simulink model "chap05"  (R2021a)
settings: Solver=FixedStepDiscrete  StartTime=0.0  StopTime=inf  FixedStep=0.001  RelTol=1e-3
undefined symbols (not defined in the file): DiscIntNeverNeededParam, Header, Pose, X, Y, Z
libraries: robotlib x31
(part 3 of 9)

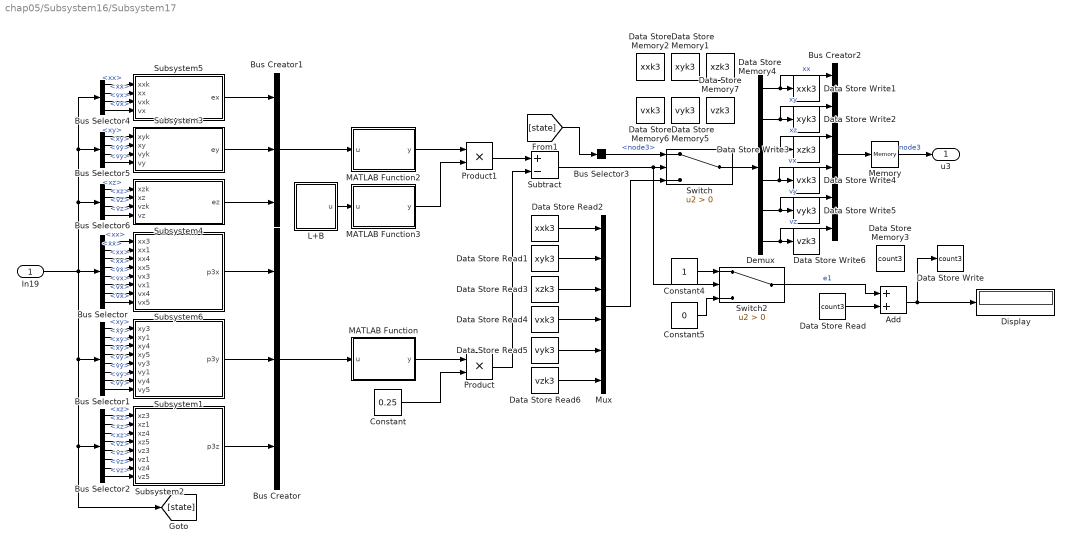
== system chap05/Subsystem16/Subsystem17 ==
  In19 : Inport
  Add : Sum
  Bus Creator : BusCreator  Inputs=3
  Bus Creator1 : BusCreator  Inputs=3
  Bus Creator2 : BusCreator  Inputs=6
  Bus Selector : BusSelector  OutputSignals=state(tk).node3.xx,state(tk).node1.xx,state(tk).node4.xx,state(tk).node5.xx,state(tk).node3.vx,state(tk).node1.vx,state(tk).node4.vx,state(tk).node5.vx
  Bus Selector1 : BusSelector  OutputSignals=state(tk).node3.xy,state(tk).node1.xy,state(tk).node4.xy,state(tk).node5.xy,state(tk).node3.vy,state(tk).node1.vy,state(tk).node4.vy,state(tk).node5.vy
  Bus Selector2 : BusSelector  OutputSignals=state(tk).node3.xz,state(tk).node1.xz,state(tk).node4.xz,state(tk).node5.xz,state(tk).node3.vz,state(tk).node1.vz,state(tk).node4.vz,state(tk).node5.vz
  Bus Selector3 : BusSelector  OutputSignals=state(t).node3
  Bus Selector4 : BusSelector  OutputSignals=state(tk).node3.xx,state(t).node3.xx,state(tk).node3.vx,state(t).node3.vx
  Bus Selector5 : BusSelector  OutputSignals=state(tk).node3.xy,state(t).node3.xy,state(tk).node3.vy,state(t).node3.vy
  Bus Selector6 : BusSelector  OutputSignals=state(tk).node3.xz,state(t).node3.xz,state(tk).node3.vz,state(t).node3.vz
  Constant : Constant  Value=0.25
  Constant4 : Constant
  Constant5 : Constant  Value=0
  Data Store Memory1 : DataStoreMemory  DataStoreName=xyk3  ReadBeforeWriteMsg=warning  WriteAfterWriteMsg=warning  WriteAfterReadMsg=warning  ShowAdditionalParam=off
  Data Store Memory2 : DataStoreMemory  DataStoreName=xxk3  ReadBeforeWriteMsg=warning  WriteAfterWriteMsg=warning  WriteAfterReadMsg=warning  ShowAdditionalParam=off
  Data Store Memory3 : DataStoreMemory  DataStoreName=count3  ReadBeforeWriteMsg=warning  WriteAfterWriteMsg=warning  WriteAfterReadMsg=warning  ShowAdditionalParam=off
  Data Store Memory4 : DataStoreMemory  DataStoreName=xzk3  ReadBeforeWriteMsg=warning  WriteAfterWriteMsg=warning  WriteAfterReadMsg=warning  ShowAdditionalParam=off
  Data Store Memory5 : DataStoreMemory  DataStoreName=vyk3  ReadBeforeWriteMsg=warning  WriteAfterWriteMsg=warning  WriteAfterReadMsg=warning  ShowAdditionalParam=off
  Data Store Memory6 : DataStoreMemory  DataStoreName=vxk3  ReadBeforeWriteMsg=warning  WriteAfterWriteMsg=warning  WriteAfterReadMsg=warning  ShowAdditionalParam=off
  Data Store Memory7 : DataStoreMemory  DataStoreName=vzk3  ReadBeforeWriteMsg=warning  WriteAfterWriteMsg=warning  WriteAfterReadMsg=warning  ShowAdditionalParam=off
  Data Store Read : DataStoreRead  DataStoreName=count3  IndexOptions=Index vector (dialog)  Indices=1  OutputSizes=1
  Data Store Read1 : DataStoreRead  DataStoreName=xyk3  IndexOptions=Index vector (dialog)  Indices=1  OutputSizes=1
  Data Store Read2 : DataStoreRead  DataStoreName=xxk3  IndexOptions=Index vector (dialog)  Indices=1  OutputSizes=1
  Data Store Read3 : DataStoreRead  DataStoreName=xzk3  IndexOptions=Index vector (dialog)  Indices=1  OutputSizes=1
  Data Store Read4 : DataStoreRead  DataStoreName=vxk3  IndexOptions=Index vector (dialog)  Indices=1  OutputSizes=1
  Data Store Read5 : DataStoreRead  DataStoreName=vyk3  IndexOptions=Index vector (dialog)  Indices=1  OutputSizes=1
  Data Store Read6 : DataStoreRead  DataStoreName=vzk3  IndexOptions=Index vector (dialog)  Indices=1  OutputSizes=1
  Data Store Write : DataStoreWrite  DataStoreName=count3  IndexOptions=Index vector (dialog)  Indices=1  OutputSizes=1
  Data Store Write1 : DataStoreWrite  DataStoreName=xxk3  IndexOptions=Index vector (dialog)  Indices=1  OutputSizes=1
  Data Store Write2 : DataStoreWrite  DataStoreName=xyk3  IndexOptions=Index vector (dialog)  Indices=1  OutputSizes=1
  Data Store Write3 : DataStoreWrite  DataStoreName=xzk3  IndexOptions=Index vector (dialog)  Indices=1  OutputSizes=1
  Data Store Write4 : DataStoreWrite  DataStoreName=vxk3  IndexOptions=Index vector (dialog)  Indices=1  OutputSizes=1
  Data Store Write5 : DataStoreWrite  DataStoreName=vyk3  IndexOptions=Index vector (dialog)  Indices=1  OutputSizes=1
  Data Store Write6 : DataStoreWrite  DataStoreName=vzk3  IndexOptions=Index vector (dialog)  Indices=1  OutputSizes=1
  Demux : Demux  Outputs=6
  Display : Display
  L+B : Subsystem
  MATLAB Function : MATLAB Function  TreatAsAtomicUnit=on
  MATLAB Function2 : MATLAB Function  TreatAsAtomicUnit=on
  MATLAB Function3 : MATLAB Function  TreatAsAtomicUnit=on
  Memory : Memory
  Mux : Mux  Inputs=6
  Product : Product
  Product1 : Product
  Subsystem1 : Subsystem
  Subsystem2 : Subsystem
  Subsystem3 : Subsystem
  Subsystem4 : Subsystem
  Subsystem5 : Subsystem
  Subsystem6 : Subsystem
  Subtract : Sum  Inputs=+-
  Switch : Switch  Criteria=u2 > Threshold
  Switch2 : Switch  Criteria=u2 > Threshold
  u3 : Outport
  wires:
  Bus Selector2/8 -> Subsystem2/8(vz5)  "<vz>"
  Bus Selector2/7 -> Subsystem2/7(vz4)  "<vz>"
  Bus Selector2/6 -> Subsystem2/6(vz1)  "<vz>"
  Bus Selector2/5 -> Subsystem2/5(vz3)  "<vz>"
  Bus Selector2/4 -> Subsystem2/4(xz5)  "<xz>"
  Bus Selector2/3 -> Subsystem2/3(xz4)  "<xz>"
  Bus Selector2/2 -> Subsystem2/2(xz1)  "<xz>"
  Bus Selector2/1 -> Subsystem2/1(xz3)  "<xz>"
  Bus Selector1/8 -> Subsystem1/8(vy5)  "<vy>"
  Bus Selector1/7 -> Subsystem1/7(vy4)  "<vy>"
  Bus Selector1/6 -> Subsystem1/6(vy1)  "<vy>"
  Bus Selector1/5 -> Subsystem1/5(vy3)  "<vy>"
  Bus Selector1/4 -> Subsystem1/4(xy5)  "<xy>"
  Bus Selector1/3 -> Subsystem1/3(xy4)  "<xy>"
  Bus Selector1/2 -> Subsystem1/2(xy1)  "<xy>"
  Bus Selector1/1 -> Subsystem1/1(xy3)  "<xy>"
  Bus Selector/8 -> Subsystem6/8(vx5)  "<vx>"
  Bus Selector/7 -> Subsystem6/7(vx4)  "<vx>"
  Bus Selector/6 -> Subsystem6/6(vx1)  "<vx>"
  Bus Selector/5 -> Subsystem6/5(vx3)  "<vx>"
  Bus Selector/4 -> Subsystem6/4(xx5)  "<xx>"
  Bus Selector/3 -> Subsystem6/3(xx4)  "<xx>"
  Bus Selector/2 -> Subsystem6/2(xx1)  "<xx>"
  Bus Selector/1 -> Subsystem6/1(xx3)  "<xx>"
  Subsystem1/1(p3y) -> Bus Creator/2
  Subsystem6/1(p3x) -> Bus Creator/1
  Subsystem2/1(p3z) -> Bus Creator/3
  Data Store Read6/1 -> Mux/6
  Switch/1 -> Demux/1
  Demux/2 -> Bus Creator2/2, Data Store Write2/1  "xy"
  Bus Selector3/1 -> Switch/1  "<node3>"
  Demux/1 -> Bus Creator2/1, Data Store Write1/1  "xx"
  Switch2/1 -> Add/1  "e1"
  Demux/6 -> Bus Creator2/6, Data Store Write6/1  "vz"
  Demux/3 -> Bus Creator2/3, Data Store Write3/1  "xz"
  Data Store Read2/1 -> Mux/1
  Constant4/1 -> Switch2/1
  Mux/1 -> Switch/3
  Data Store Read3/1 -> Mux/3
  Add/1 -> Data Store Write/1, Display/1
  Demux/4 -> Bus Creator2/4, Data Store Write4/1  "vx"
  Memory/1 -> u3/1  "node3"
  Data Store Read5/1 -> Mux/5
  Data Store Read4/1 -> Mux/4
  Product/1 -> Subtract/2
  Data Store Read1/1 -> Mux/2
  [state] -> Bus Selector3/1
  MATLAB Function3/1(y) -> Product1/2
  Bus Creator1/1 -> MATLAB Function2/1(u)
  Constant5/1 -> Switch2/3
  Constant/1 -> Product/2
  MATLAB Function2/1(y) -> Product1/1
  Subsystem4/1(ez) -> Bus Creator1/3
  Subsystem5/1(ex) -> Bus Creator1/1
  Subsystem3/1(ey) -> Bus Creator1/2
  Demux/5 -> Bus Creator2/5, Data Store Write5/1  "vy"
  Product1/1 -> Subtract/1
  Data Store Read/1 -> Add/2
  MATLAB Function/1(y) -> Product/1
  Bus Creator/1 -> MATLAB Function/1(u)
  Bus Selector6/4 -> Subsystem4/4(vz)  "<vz>"
  Bus Selector6/2 -> Subsystem4/2(xz)  "<xz>"
  Bus Selector6/3 -> Subsystem4/3(vzk)  "<vz>"
  Bus Selector6/1 -> Subsystem4/1(xzk)  "<xz>"
  Bus Selector5/3 -> Subsystem3/3(vyk)  "<vy>"
  Bus Selector5/2 -> Subsystem3/2(xy)  "<xy>"
  Bus Selector5/4 -> Subsystem3/4(vy)  "<vy>"
  Bus Selector5/1 -> Subsystem3/1(xyk)  "<xy>"
  In19/1 -> [state], Bus Selector2/1, Bus Selector1/1, Bus Selector/1, Bus Selector6/1, Bus Selector5/1, Bus Selector4/1
  Bus Selector4/1 -> Subsystem5/1(xxk)  "<xx>"
  Bus Selector4/2 -> Subsystem5/2(xx)  "<xx>"
  Bus Selector4/3 -> Subsystem5/3(vxk)  "<vx>"
  Bus Selector4/4 -> Subsystem5/4(vx)  "<vx>"
  Bus Creator2/1 -> Memory/1
  Subtract/1 -> Switch/2, Switch2/2
  L+B/1(u) -> MATLAB Function3/1(u)

== system chap05/Subsystem16/Subsystem2 ==
  In19 : Inport
  switch : Inport  Port=2
  Bus Creator : BusCreator  Inputs=3
  Bus Selector : BusSelector  OutputSignals=state(tk).node2.xx,state(tk).node1.xx,state(tk).node4.xx,state(tk).node6.xx,state(tk).node2.vx,state(tk).node1.vx,state(tk).node4.vx,state(tk).node6.vx
  Bus Selector1 : BusSelector  OutputSignals=state(tk).node2.xy,state(tk).node1.xy,state(tk).node4.xy,state(tk).node6.xy,state(tk).node2.vy,state(tk).node1.vy,state(tk).node4.vy,state(tk).node6.vy
  Bus Selector2 : BusSelector  OutputSignals=state(tk).node2.xz,state(tk).node1.xz,state(tk).node4.xz,state(tk).node6.xz,state(tk).node2.vz,state(tk).node1.vz,state(tk).node4.vz,state(tk).node6.vz
  Bus Selector3 : BusSelector  OutputSignals=state(t).node2.vx
  Bus Selector4 : BusSelector  OutputSignals=state(t).node2.vy
  Bus Selector5 : BusSelector  OutputSignals=state(t).node2.vz
  Bus Selector6 : BusSelector  OutputSignals=state(t).node2.vx,state(t).node2.vy,state(t).node2.vz
  Bus Selector7 : BusSelector  OutputSignals=state(t).node2.vx,state(t).node2.vy,state(t).node2.vz
  Bus Selector8 : BusSelector  OutputSignals=control.node2.ux,control.node2.uy,control.node2.uz
  Subsystem1 : Subsystem
  Subsystem10 : Subsystem
  Subsystem11 : Subsystem
      settings: PortSchema="{\"entries\":[{\"content\":{\"sides\":[{\"content\":{\"connectorIds\":[\"In1\",\"In2\",\"In3\"]},\"type\":\"ConnectorPlacement.EquallySpacedRectSide\",\"uuid\":\"3c32f130-2df4-4697-80e9-267a8217898e\"},{\"content\":{\"connectorIds\":[\"Out1\"],\"side\":\"RIGHT\"},\"type\":\"ConnectorPlacement.EquallySpacedRectSide\",\"uuid\":\"840675a7-4714-440f-a6ce-75eff1b2763f\"},{\"content\":{\"connectorIds\":[\"In4\"],\"side\":\"TOP\"},\"type\":\"ConnectorPlacement.EquallySpacedRectSide\",\"uuid\":\"5c23af56-4ec3-4a39-a531-12998a0be3c8\"},{\"content\":{\"connectorIds\":[\"Out2\"],\"side\":\"BOTTOM\"},\"type\":\"ConnectorPlacement.EquallySpacedRectSide\",\"uuid\":\"31d953fb-65a0-42e9-a844-060de010f298\"}]},\"type\":\"ConnectorPlacement.EquallySpacedConnector\",\"uuid\":\"61b27aa3-5880-401e-bae3-4611093a191a\"}],\"packageUris\":[\"http://schema.mathworks.com/mf0/Connector/R2020b\"],\"version\":\"1.0\"}"
  Subsystem2 : Subsystem
  Subsystem3 : Subsystem
      settings: PortSchema="{\"entries\":[{\"content\":{\"sides\":[{\"content\":{\"connectorIds\":[\"In1\",\"In2\",\"In3\",\"In4\",\"In5\",\"In6\",\"In7\",\"In8\",\"In9\"]},\"type\":\"ConnectorPlacement.EquallySpacedRectSide\",\"uuid\":\"e02b19dc-feca-4a5f-b0a9-7b682689d3dc\"},{\"content\":{\"connectorIds\":[\"Out1\",\"Out2\",\"Out3\"],\"side\":\"RIGHT\"},\"type\":\"ConnectorPlacement.EquallySpacedRectSide\",\"uuid\":\"6cba16a1-1866-4332-a766-c6ecae75c00a\"},{\"content\":{\"connectorIds\":[],\"side\":\"TOP\"},\"type\":\"ConnectorPlacement.EquallySpacedRectSide\",\"uuid\":\"834934d8-ba7c-4cfc-8528-dda956d123e9\"},{\"content\":{\"connectorIds\":[\"In10\"],\"side\":\"BOTTOM\"},\"type\":\"ConnectorPlacement.EquallySpacedRectSide\",\"uuid\":\"a447ec2e-850c-49d1-98c5-4201d925b22c\"}]},\"type\":\"ConnectorPlacement.EquallySpacedConnector\",\"uuid\":\"dde62e81-0b86-43c6-8cdc-67ebf109c079\"}],\"packageUris\":[\"http://schema.mathworks.com/mf0/Connector/R2020b\"],\"version\":\"1.0\"}"
  Subsystem4 : Subsystem
      settings: PortSchema="{\"entries\":[{\"content\":{\"sides\":[{\"content\":{\"connectorIds\":[\"In1\",\"In2\",\"In3\"]},\"type\":\"ConnectorPlacement.EquallySpacedRectSide\",\"uuid\":\"3c32f130-2df4-4697-80e9-267a8217898e\"},{\"content\":{\"connectorIds\":[\"Out1\"],\"side\":\"RIGHT\"},\"type\":\"ConnectorPlacement.EquallySpacedRectSide\",\"uuid\":\"840675a7-4714-440f-a6ce-75eff1b2763f\"},{\"content\":{\"connectorIds\":[\"In4\"],\"side\":\"TOP\"},\"type\":\"ConnectorPlacement.EquallySpacedRectSide\",\"uuid\":\"5c23af56-4ec3-4a39-a531-12998a0be3c8\"},{\"content\":{\"connectorIds\":[\"Out2\"],\"side\":\"BOTTOM\"},\"type\":\"ConnectorPlacement.EquallySpacedRectSide\",\"uuid\":\"31d953fb-65a0-42e9-a844-060de010f298\"}]},\"type\":\"ConnectorPlacement.EquallySpacedConnector\",\"uuid\":\"61b27aa3-5880-401e-bae3-4611093a191a\"}],\"packageUris\":[\"http://schema.mathworks.com/mf0/Connector/R2020b\"],\"version\":\"1.0\"}"
  Subsystem6 : Subsystem
  Subsystem8 : Subsystem
      settings: PortSchema="{\"entries\":[{\"content\":{\"sides\":[{\"content\":{\"connectorIds\":[\"In1\",\"In2\",\"In3\",\"In4\",\"In5\",\"In6\"]},\"type\":\"ConnectorPlacement.EquallySpacedRectSide\",\"uuid\":\"6e2ae49e-f829-4a88-ba6d-12a1c984ff97\"},{\"content\":{\"connectorIds\":[\"Out1\"],\"side\":\"RIGHT\"},\"type\":\"ConnectorPlacement.EquallySpacedRectSide\",\"uuid\":\"1d02df48-94d5-4b75-9fdc-37bb62799324\"},{\"content\":{\"connectorIds\":[],\"side\":\"TOP\"},\"type\":\"ConnectorPlacement.EquallySpacedRectSide\",\"uuid\":\"e0c2a01b-94eb-432a-818f-b3ac4af71c3e\"},{\"content\":{\"connectorIds\":[\"In7\"],\"side\":\"BOTTOM\"},\"type\":\"ConnectorPlacement.EquallySpacedRectSide\",\"uuid\":\"1c8c54e5-1608-4962-a210-31f0a1951aa9\"}]},\"type\":\"ConnectorPlacement.EquallySpacedConnector\",\"uuid\":\"4e183442-7783-4f10-aa1a-c21f2f9b268a\"}],\"packageUris\":[\"http://schema.mathworks.com/mf0/Connector/R2020b\"],\"version\":\"1.0\"}"
  Subsystem9 : Subsystem
      settings: PortSchema="{\"entries\":[{\"content\":{\"sides\":[{\"content\":{\"connectorIds\":[\"In1\",\"In2\",\"In3\"]},\"type\":\"ConnectorPlacement.EquallySpacedRectSide\",\"uuid\":\"3c32f130-2df4-4697-80e9-267a8217898e\"},{\"content\":{\"connectorIds\":[\"Out1\"],\"side\":\"RIGHT\"},\"type\":\"ConnectorPlacement.EquallySpacedRectSide\",\"uuid\":\"840675a7-4714-440f-a6ce-75eff1b2763f\"},{\"content\":{\"connectorIds\":[\"In4\"],\"side\":\"TOP\"},\"type\":\"ConnectorPlacement.EquallySpacedRectSide\",\"uuid\":\"5c23af56-4ec3-4a39-a531-12998a0be3c8\"},{\"content\":{\"connectorIds\":[\"Out2\"],\"side\":\"BOTTOM\"},\"type\":\"ConnectorPlacement.EquallySpacedRectSide\",\"uuid\":\"31d953fb-65a0-42e9-a844-060de010f298\"}]},\"type\":\"ConnectorPlacement.EquallySpacedConnector\",\"uuid\":\"61b27aa3-5880-401e-bae3-4611093a191a\"}],\"packageUris\":[\"http://schema.mathworks.com/mf0/Connector/R2020b\"],\"version\":\"1.0\"}"
  u2 : Outport
  wires:
  Bus Creator/1 -> u2/1  "node2"
  Bus Selector6/1 -> Subsystem8/4(vx)  "<vx>"
  Bus Selector6/2 -> Subsystem8/5(vy)  "<vy>"
  Bus Selector6/3 -> Subsystem8/6(vz)  "<vz>"
  [Sz] -> Subsystem8/3(Sz)
  [Sx] -> Subsystem8/1(Sx)
  [state] -> Bus Selector6/1
  [Sy] -> Subsystem8/2(Sy)
  Subsystem8/1(" gain") -> [gain]  "p2"
  Subsystem10/1(ux) -> Bus Creator/1  "ux"
  Subsystem10/2(uy) -> Bus Creator/2  "uy"
  Subsystem10/3(uz) -> Bus Creator/3  "uz"
  Bus Selector8/3 -> Subsystem3/8(uz)  "<uz>"
  Bus Selector7/3 -> Subsystem3/4(vz)  "<vz>"
  Bus Selector7/2 -> Subsystem3/3(vy)  "<vy>"
  Bus Selector7/1 -> Subsystem3/2(vx)  "<vx>"
  Bus Selector8/1 -> Subsystem3/6(ux)  "<ux>"
  [state] -> Bus Selector7/1
  Bus Selector8/2 -> Subsystem3/7(uy)  "<uy>"
  [state] -> Bus Selector8/1
  Subsystem3/1(udtx) -> Subsystem10/1(utx)
  Subsystem3/2(udty) -> Subsystem10/2(uty)
  Subsystem3/3(udtz) -> Subsystem10/3(utz)
  Subsystem11/2(Sz) -> [Sz]
  Subsystem9/1(uy) -> Subsystem3/5(uty)
  Subsystem1/1(p2y) -> Subsystem9/2(uty)
  [state] -> Bus Selector4/1
  Subsystem4/1(ux) -> Subsystem3/1(utx)
  Subsystem2/1(p2z) -> Subsystem11/2(utz)
  Bus Selector4/1 -> Subsystem9/1(vy2)  "<vy>"
  Bus Selector5/1 -> Subsystem11/1(vz2)  "<vz>"
  [gain] -> Subsystem11/3(gain)
  [gain] -> Subsystem4/3(gain)
  Subsystem11/1(uz) -> Subsystem3/9(utz)
  [gain] -> Subsystem9/3(gain)
  [state] -> Bus Selector3/1
  Subsystem6/1(p2x) -> Subsystem4/2(utx)
  Subsystem9/2(Sz) -> [Sy]
  Bus Selector3/1 -> Subsystem4/1(vx2)  "<vx>"
  Subsystem4/2(Sx) -> [Sx]
  [state] -> Bus Selector5/1
  In19/1 -> [state], Bus Selector2/1, Bus Selector/1, Bus Selector1/1
  Bus Selector1/6 -> Subsystem1/6(vy1)  "<vy>"
  Bus Selector2/6 -> Subsystem2/6(vz1)  "<vz>"
  Bus Selector/7 -> Subsystem6/7(vx4)  "<vx>"
  Bus Selector/3 -> Subsystem6/3(xx4)  "<xx>"
  Bus Selector1/2 -> Subsystem1/2(xy1)  "<xy>"
  Bus Selector1/5 -> Subsystem1/5(vy2)  "<vy>"
  Bus Selector/2 -> Subsystem6/2(xx1)  "<xx>"
  Bus Selector/6 -> Subsystem6/6(vx1)  "<vx>"
  Bus Selector/8 -> Subsystem6/8(vx6)  "<vx>"
  Bus Selector1/8 -> Subsystem1/8(vy6)  "<vy>"
  Bus Selector/1 -> Subsystem6/1(xx2)  "<xx>"
  Bus Selector/5 -> Subsystem6/5(vx2)  "<vx>"
  Bus Selector1/1 -> Subsystem1/1(xy2)  "<xy>"
  Bus Selector2/3 -> Subsystem2/3(xz4)  "<xz>"
  Bus Selector2/4 -> Subsystem2/4(xz6)  "<xz>"
  Bus Selector2/5 -> Subsystem2/5(vz2)  "<vz>"
  Bus Selector2/7 -> Subsystem2/7(vz4)  "<vz>"
  Bus Selector2/1 -> Subsystem2/1(xz2)  "<xz>"
  Bus Selector2/2 -> Subsystem2/2(xz1)  "<xz>"
  Bus Selector1/7 -> Subsystem1/7(vy4)  "<vy>"
  Bus Selector1/3 -> Subsystem1/3(xy4)  "<xy>"
  Bus Selector1/4 -> Subsystem1/4(xy6)  "<xy>"
  Bus Selector/4 -> Subsystem6/4(xx6)  "<xx>"
  Bus Selector2/8 -> Subsystem2/8(vz6)  "<vz>"
  switch/1 -> [switch], Subsystem4/4(switch)
  [switch] -> Subsystem9/4(switch)
  [switch] -> Subsystem11/4(switch)
  [switch] -> Subsystem3/10(switch)
  [switch] -> Subsystem8/7(switch)

== system chap05/Subsystem16/Subsystem3 ==
  In19 : Inport
  switch : Inport  Port=2
  Bus Creator : BusCreator  Inputs=3
  Bus Selector : BusSelector  OutputSignals=state(tk).node4.xx,state(tk).node2.xx,state(tk).node3.xx,state(tk).node5.xx,state(tk).node4.vx,state(tk).node2.vx,state(tk).node3.vx,state(tk).node5.vx
  Bus Selector1 : BusSelector  OutputSignals=state(tk).node4.xy,state(tk).node2.xy,state(tk).node3.xy,state(tk).node5.xy,state(tk).node4.vy,state(tk).node2.vy,state(tk).node3.vy,state(tk).node5.vy
  Bus Selector2 : BusSelector  OutputSignals=state(tk).node4.xz,state(tk).node2.xz,state(tk).node3.xz,state(tk).node5.xz,state(tk).node4.vz,state(tk).node2.vz,state(tk).node3.vz,state(tk).node5.vz
  Bus Selector3 : BusSelector  OutputSignals=state(t).node4.vx
  Bus Selector4 : BusSelector  OutputSignals=state(t).node4.vy
  Bus Selector5 : BusSelector  OutputSignals=state(t).node4.vz
  Bus Selector6 : BusSelector  OutputSignals=state(t).node4.vx,state(t).node4.vy,state(t).node4.vz
  Bus Selector7 : BusSelector  OutputSignals=state(t).node4.vx,state(t).node4.vy,state(t).node4.vz
  Bus Selector8 : BusSelector  OutputSignals=control.node4.ux,control.node4.uy,control.node4.uz
  Subsystem1 : Subsystem
  Subsystem10 : Subsystem
  Subsystem11 : Subsystem
      settings: PortSchema="{\"entries\":[{\"content\":{\"sides\":[{\"content\":{\"connectorIds\":[\"In1\",\"In2\",\"In3\"]},\"type\":\"ConnectorPlacement.EquallySpacedRectSide\",\"uuid\":\"3c32f130-2df4-4697-80e9-267a8217898e\"},{\"content\":{\"connectorIds\":[\"Out1\"],\"side\":\"RIGHT\"},\"type\":\"ConnectorPlacement.EquallySpacedRectSide\",\"uuid\":\"840675a7-4714-440f-a6ce-75eff1b2763f\"},{\"content\":{\"connectorIds\":[\"In4\"],\"side\":\"TOP\"},\"type\":\"ConnectorPlacement.EquallySpacedRectSide\",\"uuid\":\"5c23af56-4ec3-4a39-a531-12998a0be3c8\"},{\"content\":{\"connectorIds\":[\"Out2\"],\"side\":\"BOTTOM\"},\"type\":\"ConnectorPlacement.EquallySpacedRectSide\",\"uuid\":\"31d953fb-65a0-42e9-a844-060de010f298\"}]},\"type\":\"ConnectorPlacement.EquallySpacedConnector\",\"uuid\":\"61b27aa3-5880-401e-bae3-4611093a191a\"}],\"packageUris\":[\"http://schema.mathworks.com/mf0/Connector/R2020b\"],\"version\":\"1.0\"}"
  Subsystem2 : Subsystem
  Subsystem3 : Subsystem
      settings: PortSchema="{\"entries\":[{\"content\":{\"sides\":[{\"content\":{\"connectorIds\":[\"In1\",\"In2\",\"In3\",\"In4\",\"In5\",\"In6\",\"In7\",\"In8\",\"In9\"]},\"type\":\"ConnectorPlacement.EquallySpacedRectSide\",\"uuid\":\"e02b19dc-feca-4a5f-b0a9-7b682689d3dc\"},{\"content\":{\"connectorIds\":[\"Out1\",\"Out2\",\"Out3\"],\"side\":\"RIGHT\"},\"type\":\"ConnectorPlacement.EquallySpacedRectSide\",\"uuid\":\"6cba16a1-1866-4332-a766-c6ecae75c00a\"},{\"content\":{\"connectorIds\":[],\"side\":\"TOP\"},\"type\":\"ConnectorPlacement.EquallySpacedRectSide\",\"uuid\":\"834934d8-ba7c-4cfc-8528-dda956d123e9\"},{\"content\":{\"connectorIds\":[\"In10\"],\"side\":\"BOTTOM\"},\"type\":\"ConnectorPlacement.EquallySpacedRectSide\",\"uuid\":\"a447ec2e-850c-49d1-98c5-4201d925b22c\"}]},\"type\":\"ConnectorPlacement.EquallySpacedConnector\",\"uuid\":\"dde62e81-0b86-43c6-8cdc-67ebf109c079\"}],\"packageUris\":[\"http://schema.mathworks.com/mf0/Connector/R2020b\"],\"version\":\"1.0\"}"
  Subsystem4 : Subsystem
      settings: PortSchema="{\"entries\":[{\"content\":{\"sides\":[{\"content\":{\"connectorIds\":[\"In1\",\"In2\",\"In3\"]},\"type\":\"ConnectorPlacement.EquallySpacedRectSide\",\"uuid\":\"3c32f130-2df4-4697-80e9-267a8217898e\"},{\"content\":{\"connectorIds\":[\"Out1\"],\"side\":\"RIGHT\"},\"type\":\"ConnectorPlacement.EquallySpacedRectSide\",\"uuid\":\"840675a7-4714-440f-a6ce-75eff1b2763f\"},{\"content\":{\"connectorIds\":[\"In4\"],\"side\":\"TOP\"},\"type\":\"ConnectorPlacement.EquallySpacedRectSide\",\"uuid\":\"5c23af56-4ec3-4a39-a531-12998a0be3c8\"},{\"content\":{\"connectorIds\":[\"Out2\"],\"side\":\"BOTTOM\"},\"type\":\"ConnectorPlacement.EquallySpacedRectSide\",\"uuid\":\"31d953fb-65a0-42e9-a844-060de010f298\"}]},\"type\":\"ConnectorPlacement.EquallySpacedConnector\",\"uuid\":\"61b27aa3-5880-401e-bae3-4611093a191a\"}],\"packageUris\":[\"http://schema.mathworks.com/mf0/Connector/R2020b\"],\"version\":\"1.0\"}"
  Subsystem6 : Subsystem
  Subsystem8 : Subsystem
      settings: PortSchema="{\"entries\":[{\"content\":{\"sides\":[{\"content\":{\"connectorIds\":[\"In1\",\"In2\",\"In3\",\"In4\",\"In5\",\"In6\"]},\"type\":\"ConnectorPlacement.EquallySpacedRectSide\",\"uuid\":\"6e2ae49e-f829-4a88-ba6d-12a1c984ff97\"},{\"content\":{\"connectorIds\":[\"Out1\"],\"side\":\"RIGHT\"},\"type\":\"ConnectorPlacement.EquallySpacedRectSide\",\"uuid\":\"1d02df48-94d5-4b75-9fdc-37bb62799324\"},{\"content\":{\"connectorIds\":[],\"side\":\"TOP\"},\"type\":\"ConnectorPlacement.EquallySpacedRectSide\",\"uuid\":\"e0c2a01b-94eb-432a-818f-b3ac4af71c3e\"},{\"content\":{\"connectorIds\":[\"In7\"],\"side\":\"BOTTOM\"},\"type\":\"ConnectorPlacement.EquallySpacedRectSide\",\"uuid\":\"1c8c54e5-1608-4962-a210-31f0a1951aa9\"}]},\"type\":\"ConnectorPlacement.EquallySpacedConnector\",\"uuid\":\"4e183442-7783-4f10-aa1a-c21f2f9b268a\"}],\"packageUris\":[\"http://schema.mathworks.com/mf0/Connector/R2020b\"],\"version\":\"1.0\"}"
  Subsystem9 : Subsystem
      settings: PortSchema="{\"entries\":[{\"content\":{\"sides\":[{\"content\":{\"connectorIds\":[\"In1\",\"In2\",\"In3\"]},\"type\":\"ConnectorPlacement.EquallySpacedRectSide\",\"uuid\":\"3c32f130-2df4-4697-80e9-267a8217898e\"},{\"content\":{\"connectorIds\":[\"Out1\"],\"side\":\"RIGHT\"},\"type\":\"ConnectorPlacement.EquallySpacedRectSide\",\"uuid\":\"840675a7-4714-440f-a6ce-75eff1b2763f\"},{\"content\":{\"connectorIds\":[\"In4\"],\"side\":\"TOP\"},\"type\":\"ConnectorPlacement.EquallySpacedRectSide\",\"uuid\":\"5c23af56-4ec3-4a39-a531-12998a0be3c8\"},{\"content\":{\"connectorIds\":[\"Out2\"],\"side\":\"BOTTOM\"},\"type\":\"ConnectorPlacement.EquallySpacedRectSide\",\"uuid\":\"31d953fb-65a0-42e9-a844-060de010f298\"}]},\"type\":\"ConnectorPlacement.EquallySpacedConnector\",\"uuid\":\"61b27aa3-5880-401e-bae3-4611093a191a\"}],\"packageUris\":[\"http://schema.mathworks.com/mf0/Connector/R2020b\"],\"version\":\"1.0\"}"
  u4 : Outport
  wires:
  Bus Creator/1 -> u4/1  "node4"
  Bus Selector/2 -> Subsystem6/2(xx2)  "<xx>"
  Bus Selector1/7 -> Subsystem1/7(vy3)  "<vy>"
  Bus Selector1/4 -> Subsystem1/4(xy5)  "<xy>"
  Bus Selector2/3 -> Subsystem2/3(xz3)  "<xz>"
  Bus Selector/8 -> Subsystem6/8(vx5)  "<vx>"
  Bus Selector2/2 -> Subsystem2/2(xx2)  "<xz>"
  Bus Selector2/4 -> Subsystem2/4(xz5)  "<xz>"
  Bus Selector1/5 -> Subsystem1/5(vy4)  "<vy>"
  Bus Selector1/2 -> Subsystem1/2(xy2)  "<xy>"
  Bus Selector2/7 -> Subsystem2/7(vz3)  "<vz>"
  Bus Selector2/5 -> Subsystem2/5(vz4)  "<vz>"
  Bus Selector1/6 -> Subsystem1/6(vy2)  "<vy>"
  Bus Selector2/8 -> Subsystem2/8(vz5)  "<vz>"
  Bus Selector2/6 -> Subsystem2/6(vz2)  "<vz>"
  Bus Selector1/3 -> Subsystem1/3(xy3)  "<xy>"
  Bus Selector2/1 -> Subsystem2/1(xz4)  "<xz>"
  Bus Selector/5 -> Subsystem6/5(vx4)  "<vx>"
  Bus Selector/1 -> Subsystem6/1(xx4)  "<xx>"
  Bus Selector/3 -> Subsystem6/3(xx3)  "<xx>"
  Bus Selector1/8 -> Subsystem1/8(vy5)  "<vy>"
  Bus Selector1/1 -> Subsystem1/1(xy4)  "<xy>"
  Bus Selector/7 -> Subsystem6/7(vx3)  "<vx>"
  Bus Selector/6 -> Subsystem6/6(vx2)  "<vx>"
  Bus Selector/4 -> Subsystem6/4(xx5)  "<xx>"
  [state] -> Bus Selector5/1
  Subsystem2/1(utx) -> Subsystem11/2(utz)
  Bus Selector5/1 -> Subsystem11/1(vz4)  "<vz>"
  [state] -> Bus Selector4/1
  [gain] -> Subsystem11/3(gain)
  Bus Selector6/3 -> Subsystem8/6(vz)  "<vz>"
  Bus Selector6/1 -> Subsystem8/4(vx)  "<vx>"
  [Sx] -> Subsystem8/1(Sx)
  [Sz] -> Subsystem8/3(Sz)
  Subsystem8/1(" gain") -> [gain]  "p4"
  Subsystem6/1(utx) -> Subsystem4/2(utx)
  In19/1 -> [state], Bus Selector2/1, Bus Selector/1, Bus Selector1/1
  [state] -> Bus Selector6/1
  Bus Selector4/1 -> Subsystem9/1(vy4)  "<vy>"
  Subsystem1/1(utx) -> Subsystem9/2(uty)
  Bus Selector3/1 -> Subsystem4/1(vx4)  "<vx>"
  Subsystem9/2(Sz) -> [Sy]
  [gain] -> Subsystem9/3(gain)
  [Sy] -> Subsystem8/2(Sy)
  [gain] -> Subsystem4/3(gain)
  [state] -> Bus Selector3/1
  Subsystem11/2(Sz) -> [Sz]
  Bus Selector6/2 -> Subsystem8/5(vy)  "<vy>"
  Subsystem4/2(Sx) -> [Sx]
  Subsystem10/1(ux) -> Bus Creator/1  "ux"
  Subsystem10/2(uy) -> Bus Creator/2  "uy"
  Subsystem10/3(uz) -> Bus Creator/3  "uz"
  Subsystem4/1(ux) -> Subsystem3/1(utx)
  Subsystem9/1(uy) -> Subsystem3/5(uty)
  Subsystem11/1(uz) -> Subsystem3/9(utz)
  [state] -> Bus Selector7/1
  Bus Selector8/1 -> Subsystem3/6(ux)  "<ux>"
  Bus Selector7/2 -> Subsystem3/3(vy)  "<vy>"
  Bus Selector8/2 -> Subsystem3/7(uy)  "<uy>"
  [state] -> Bus Selector8/1
  Bus Selector7/1 -> Subsystem3/2(vx)  "<vx>"
  Bus Selector7/3 -> Subsystem3/4(vz)  "<vz>"
  Bus Selector8/3 -> Subsystem3/8(uz)  "<uz>"
  Subsystem3/1(udtx) -> Subsystem10/1(utx)
  Subsystem3/2(udty) -> Subsystem10/2(uty)
  Subsystem3/3(udtz) -> Subsystem10/3(utz)
  [switch] -> Subsystem8/7(switch)
  switch/1 -> [switch], Subsystem4/4(switch)
  [switch] -> Subsystem11/4(switch)
  [switch] -> Subsystem9/4(switch)
  [switch] -> Subsystem3/10(switch)

== system chap05/Subsystem16/Subsystem5 ==
  In19 : Inport
  switch : Inport  Port=2
  Bus Creator : BusCreator  Inputs=3
  Bus Selector : BusSelector  OutputSignals=state(tk).node3.xx,state(tk).node1.xx,state(tk).node4.xx,state(tk).node5.xx,state(tk).node3.vx,state(tk).node1.vx,state(tk).node4.vx,state(tk).node5.vx
  Bus Selector1 : BusSelector  OutputSignals=state(tk).node3.xy,state(tk).node1.xy,state(tk).node4.xy,state(tk).node5.xy,state(tk).node3.vy,state(tk).node1.vy,state(tk).node4.vy,state(tk).node5.vy
  Bus Selector2 : BusSelector  OutputSignals=state(tk).node3.xz,state(tk).node1.xz,state(tk).node4.xz,state(tk).node5.xz,state(tk).node3.vz,state(tk).node1.vz,state(tk).node4.vz,state(tk).node5.vz
  Bus Selector3 : BusSelector  OutputSignals=state(t).node3.vx
  Bus Selector4 : BusSelector  OutputSignals=state(t).node3.vy
  Bus Selector5 : BusSelector  OutputSignals=state(t).node3.vz
  Bus Selector6 : BusSelector  OutputSignals=state(t).node3.vx,state(t).node3.vy,state(t).node3.vz
  Bus Selector7 : BusSelector  OutputSignals=state(t).node3.vx,state(t).node3.vy,state(t).node3.vz
  Bus Selector8 : BusSelector  OutputSignals=control.node3.ux,control.node3.uy,control.node3.uz
  Subsystem1 : Subsystem
  Subsystem10 : Subsystem
  Subsystem11 : Subsystem
      settings: PortSchema="{\"entries\":[{\"content\":{\"sides\":[{\"content\":{\"connectorIds\":[\"In1\",\"In2\",\"In3\"]},\"type\":\"ConnectorPlacement.EquallySpacedRectSide\",\"uuid\":\"3c32f130-2df4-4697-80e9-267a8217898e\"},{\"content\":{\"connectorIds\":[\"Out1\"],\"side\":\"RIGHT\"},\"type\":\"ConnectorPlacement.EquallySpacedRectSide\",\"uuid\":\"840675a7-4714-440f-a6ce-75eff1b2763f\"},{\"content\":{\"connectorIds\":[\"In4\"],\"side\":\"TOP\"},\"type\":\"ConnectorPlacement.EquallySpacedRectSide\",\"uuid\":\"5c23af56-4ec3-4a39-a531-12998a0be3c8\"},{\"content\":{\"connectorIds\":[\"Out2\"],\"side\":\"BOTTOM\"},\"type\":\"ConnectorPlacement.EquallySpacedRectSide\",\"uuid\":\"31d953fb-65a0-42e9-a844-060de010f298\"}]},\"type\":\"ConnectorPlacement.EquallySpacedConnector\",\"uuid\":\"61b27aa3-5880-401e-bae3-4611093a191a\"}],\"packageUris\":[\"http://schema.mathworks.com/mf0/Connector/R2020b\"],\"version\":\"1.0\"}"
  Subsystem2 : Subsystem
  Subsystem3 : Subsystem
      settings: PortSchema="{\"entries\":[{\"content\":{\"sides\":[{\"content\":{\"connectorIds\":[\"In1\",\"In2\",\"In3\",\"In4\",\"In5\",\"In6\",\"In7\",\"In8\",\"In9\"]},\"type\":\"ConnectorPlacement.EquallySpacedRectSide\",\"uuid\":\"e02b19dc-feca-4a5f-b0a9-7b682689d3dc\"},{\"content\":{\"connectorIds\":[\"Out1\",\"Out2\",\"Out3\"],\"side\":\"RIGHT\"},\"type\":\"ConnectorPlacement.EquallySpacedRectSide\",\"uuid\":\"6cba16a1-1866-4332-a766-c6ecae75c00a\"},{\"content\":{\"connectorIds\":[],\"side\":\"TOP\"},\"type\":\"ConnectorPlacement.EquallySpacedRectSide\",\"uuid\":\"834934d8-ba7c-4cfc-8528-dda956d123e9\"},{\"content\":{\"connectorIds\":[\"In10\"],\"side\":\"BOTTOM\"},\"type\":\"ConnectorPlacement.EquallySpacedRectSide\",\"uuid\":\"a447ec2e-850c-49d1-98c5-4201d925b22c\"}]},\"type\":\"ConnectorPlacement.EquallySpacedConnector\",\"uuid\":\"dde62e81-0b86-43c6-8cdc-67ebf109c079\"}],\"packageUris\":[\"http://schema.mathworks.com/mf0/Connector/R2020b\"],\"version\":\"1.0\"}"
  Subsystem4 : Subsystem
      settings: PortSchema="{\"entries\":[{\"content\":{\"sides\":[{\"content\":{\"connectorIds\":[\"In1\",\"In2\",\"In3\"]},\"type\":\"ConnectorPlacement.EquallySpacedRectSide\",\"uuid\":\"3c32f130-2df4-4697-80e9-267a8217898e\"},{\"content\":{\"connectorIds\":[\"Out1\"],\"side\":\"RIGHT\"},\"type\":\"ConnectorPlacement.EquallySpacedRectSide\",\"uuid\":\"840675a7-4714-440f-a6ce-75eff1b2763f\"},{\"content\":{\"connectorIds\":[\"In4\"],\"side\":\"TOP\"},\"type\":\"ConnectorPlacement.EquallySpacedRectSide\",\"uuid\":\"5c23af56-4ec3-4a39-a531-12998a0be3c8\"},{\"content\":{\"connectorIds\":[\"Out2\"],\"side\":\"BOTTOM\"},\"type\":\"ConnectorPlacement.EquallySpacedRectSide\",\"uuid\":\"31d953fb-65a0-42e9-a844-060de010f298\"}]},\"type\":\"ConnectorPlacement.EquallySpacedConnector\",\"uuid\":\"61b27aa3-5880-401e-bae3-4611093a191a\"}],\"packageUris\":[\"http://schema.mathworks.com/mf0/Connector/R2020b\"],\"version\":\"1.0\"}"
  Subsystem6 : Subsystem
  Subsystem7 : Subsystem
      settings: PortSchema="{\"entries\":[{\"content\":{\"sides\":[{\"content\":{\"connectorIds\":[\"In1\",\"In2\",\"In3\",\"In4\",\"In5\",\"In6\"]},\"type\":\"ConnectorPlacement.EquallySpacedRectSide\",\"uuid\":\"6e2ae49e-f829-4a88-ba6d-12a1c984ff97\"},{\"content\":{\"connectorIds\":[\"Out1\"],\"side\":\"RIGHT\"},\"type\":\"ConnectorPlacement.EquallySpacedRectSide\",\"uuid\":\"1d02df48-94d5-4b75-9fdc-37bb62799324\"},{\"content\":{\"connectorIds\":[],\"side\":\"TOP\"},\"type\":\"ConnectorPlacement.EquallySpacedRectSide\",\"uuid\":\"e0c2a01b-94eb-432a-818f-b3ac4af71c3e\"},{\"content\":{\"connectorIds\":[\"In7\"],\"side\":\"BOTTOM\"},\"type\":\"ConnectorPlacement.EquallySpacedRectSide\",\"uuid\":\"1c8c54e5-1608-4962-a210-31f0a1951aa9\"}]},\"type\":\"ConnectorPlacement.EquallySpacedConnector\",\"uuid\":\"4e183442-7783-4f10-aa1a-c21f2f9b268a\"}],\"packageUris\":[\"http://schema.mathworks.com/mf0/Connector/R2020b\"],\"version\":\"1.0\"}"
  Subsystem9 : Subsystem
      settings: PortSchema="{\"entries\":[{\"content\":{\"sides\":[{\"content\":{\"connectorIds\":[\"In1\",\"In2\",\"In3\"]},\"type\":\"ConnectorPlacement.EquallySpacedRectSide\",\"uuid\":\"3c32f130-2df4-4697-80e9-267a8217898e\"},{\"content\":{\"connectorIds\":[\"Out1\"],\"side\":\"RIGHT\"},\"type\":\"ConnectorPlacement.EquallySpacedRectSide\",\"uuid\":\"840675a7-4714-440f-a6ce-75eff1b2763f\"},{\"content\":{\"connectorIds\":[\"In4\"],\"side\":\"TOP\"},\"type\":\"ConnectorPlacement.EquallySpacedRectSide\",\"uuid\":\"5c23af56-4ec3-4a39-a531-12998a0be3c8\"},{\"content\":{\"connectorIds\":[\"Out2\"],\"side\":\"BOTTOM\"},\"type\":\"ConnectorPlacement.EquallySpacedRectSide\",\"uuid\":\"31d953fb-65a0-42e9-a844-060de010f298\"}]},\"type\":\"ConnectorPlacement.EquallySpacedConnector\",\"uuid\":\"61b27aa3-5880-401e-bae3-4611093a191a\"}],\"packageUris\":[\"http://schema.mathworks.com/mf0/Connector/R2020b\"],\"version\":\"1.0\"}"
  u3 : Outport
  wires:
  Bus Creator/1 -> u3/1  "node3"
  [state] -> Bus Selector6/1
  [Sz] -> Subsystem7/3(Sz)
  [Sx] -> Subsystem7/1(Sx)
  Bus Selector6/3 -> Subsystem7/6(vz)  "<vz>"
  [Sy] -> Subsystem7/2(Sy)
  Bus Selector6/1 -> Subsystem7/4(vx)  "<vx>"
  Bus Selector6/2 -> Subsystem7/5(vy)  "<vy>"
  Subsystem10/1(ux) -> Bus Creator/1  "ux"
  Subsystem10/2(uy) -> Bus Creator/2  "uy"
  Subsystem10/3(uz) -> Bus Creator/3  "uz"
  [state] -> Bus Selector7/1
  Bus Selector8/1 -> Subsystem3/6(ux)  "<ux>"
  Bus Selector7/2 -> Subsystem3/3(vy)  "<vy>"
  Bus Selector8/2 -> Subsystem3/7(uy)  "<uy>"
  [state] -> Bus Selector8/1
  Bus Selector7/1 -> Subsystem3/2(vx)  "<vx>"
  Bus Selector7/3 -> Subsystem3/4(vz)  "<vz>"
  Bus Selector8/3 -> Subsystem3/8(uz)  "<uz>"
  Subsystem3/1(udtx) -> Subsystem10/1(utx)
  Subsystem3/2(udty) -> Subsystem10/2(uty)
  Subsystem3/3(udtz) -> Subsystem10/3(utz)
  Subsystem7/1(" gain") -> [gain]  "p3"
  Bus Selector2/8 -> Subsystem2/8(vz5)  "<vz>"
  In19/1 -> Bus Selector/1, Bus Selector1/1, [state], Bus Selector2/1
  Bus Selector1/4 -> Subsystem1/4(xy5)  "<xy>"
  Bus Selector/4 -> Subsystem6/4(xx5)  "<xx>"
  Bus Selector/2 -> Subsystem6/2(xx1)  "<xx>"
  Bus Selector/1 -> Subsystem6/1(xx3)  "<xx>"
  Bus Selector/8 -> Subsystem6/8(vx5)  "<vx>"
  Bus Selector2/7 -> Subsystem2/7(vz4)  "<vz>"
  Bus Selector1/5 -> Subsystem1/5(vy3)  "<vy>"
  Bus Selector1/1 -> Subsystem1/1(xy3)  "<xy>"
  Bus Selector/3 -> Subsystem6/3(xx4)  "<xx>"
  Bus Selector/5 -> Subsystem6/5(vx3)  "<vx>"
  Bus Selector1/6 -> Subsystem1/6(vy1)  "<vy>"
  Bus Selector2/3 -> Subsystem2/3(xz4)  "<xz>"
  Bus Selector1/8 -> Subsystem1/8(vy5)  "<vy>"
  Bus Selector2/1 -> Subsystem2/1(xz3)  "<xz>"
  Bus Selector1/3 -> Subsystem1/3(xy4)  "<xy>"
  Bus Selector1/2 -> Subsystem1/2(xy1)  "<xy>"
  Bus Selector1/7 -> Subsystem1/7(vy4)  "<vy>"
  Bus Selector2/2 -> Subsystem2/2(xz1)  "<xz>"
  Bus Selector2/4 -> Subsystem2/4(xz5)  "<xz>"
  Bus Selector2/6 -> Subsystem2/6(vz1)  "<vz>"
  Bus Selector2/5 -> Subsystem2/5(vz3)  "<vz>"
  Bus Selector/7 -> Subsystem6/7(vx4)  "<vx>"
  Bus Selector/6 -> Subsystem6/6(vx1)  "<vx>"
  Subsystem6/1(p3x) -> Subsystem4/2(utx)
  [gain] -> Subsystem9/3(gain)
  Bus Selector4/1 -> Subsystem9/1(vy3)  "<vy>"
  [state] -> Bus Selector5/1
  [state] -> Bus Selector3/1
  Subsystem4/2(Sx) -> [Sx]
  Bus Selector3/1 -> Subsystem4/1(vx3)  "<vx>"
  Subsystem9/1(uy) -> Subsystem3/5(uty)
  Bus Selector5/1 -> Subsystem11/1(vz3)  "<vz>"
  [gain] -> Subsystem4/3(gain)
  Subsystem11/1(uz) -> Subsystem3/9(utz)
  [gain] -> Subsystem11/3(gain)
  Subsystem2/1(p3z) -> Subsystem11/2(utz)
  Subsystem4/1(ux) -> Subsystem3/1(utx)
  Subsystem1/1(p3y) -> Subsystem9/2(uty)
  [state] -> Bus Selector4/1
  Subsystem11/2(Sz) -> [Sz]
  Subsystem9/2(Sz) -> [Sy]
  switch/1 -> [switch], Subsystem4/4(switch)
  [switch] -> Subsystem9/4(switch)
  [switch] -> Subsystem11/4(switch)
  [switch] -> Subsystem3/10(switch)
  [switch] -> Subsystem7/7(switch)

== system chap05/Subsystem16/Subsystem6 ==
  In19 : Inport
  switch : Inport  Port=2
  Bus Creator : BusCreator  Inputs=3
  Bus Selector : BusSelector  OutputSignals=state(tk).node6.xx,state(tk).node6.xx0,state(tk).node1.xx,state(tk).node2.xx,state(tk).node6.vx,state(tk).node6.vx0,state(tk).node1.vx,state(tk).node2.vx
  Bus Selector1 : BusSelector  OutputSignals=state(tk).node6.xy,state(tk).node6.xy0,state(tk).node1.xy,state(tk).node2.xy,state(tk).node6.vy,state(tk).node6.vy0,state(tk).node1.vy,state(tk).node2.vy
  Bus Selector2 : BusSelector  OutputSignals=state(tk).node6.xz,state(tk).node6.xz0,state(tk).node1.xz,state(tk).node2.xz,state(tk).node6.vz,state(tk).node6.vz0,state(tk).node1.vz,state(tk).node2.vz
  Bus Selector3 : BusSelector  OutputSignals=state(t).node6.vx,state(t).node0.vx
  Bus Selector4 : BusSelector  OutputSignals=state(t).node6.vy,state(t).node0.vx
  Bus Selector5 : BusSelector  OutputSignals=state(t).node6.vz,state(t).node0.vz
  Bus Selector6 : BusSelector  OutputSignals=state(t).node6.vx,state(t).node6.vy,state(t).node6.vz
  Bus Selector7 : BusSelector  OutputSignals=state(t).node6.vx,state(t).node6.vy,state(t).node6.vz
  Bus Selector8 : BusSelector  OutputSignals=control.node6.ux,control.node6.uy,control.node6.uz
  Subsystem1 : Subsystem
  Subsystem10 : Subsystem
  Subsystem2 : Subsystem
  Subsystem3 : Subsystem
      settings: PortSchema="{\"entries\":[{\"content\":{\"sides\":[{\"content\":{\"connectorIds\":[\"In1\",\"In2\",\"In3\",\"In4\",\"In5\",\"In6\",\"In7\",\"In8\",\"In9\"]},\"type\":\"ConnectorPlacement.EquallySpacedRectSide\",\"uuid\":\"e02b19dc-feca-4a5f-b0a9-7b682689d3dc\"},{\"content\":{\"connectorIds\":[\"Out1\",\"Out2\",\"Out3\"],\"side\":\"RIGHT\"},\"type\":\"ConnectorPlacement.EquallySpacedRectSide\",\"uuid\":\"6cba16a1-1866-4332-a766-c6ecae75c00a\"},{\"content\":{\"connectorIds\":[],\"side\":\"TOP\"},\"type\":\"ConnectorPlacement.EquallySpacedRectSide\",\"uuid\":\"834934d8-ba7c-4cfc-8528-dda956d123e9\"},{\"content\":{\"connectorIds\":[\"In10\"],\"side\":\"BOTTOM\"},\"type\":\"ConnectorPlacement.EquallySpacedRectSide\",\"uuid\":\"a447ec2e-850c-49d1-98c5-4201d925b22c\"}]},\"type\":\"ConnectorPlacement.EquallySpacedConnector\",\"uuid\":\"dde62e81-0b86-43c6-8cdc-67ebf109c079\"}],\"packageUris\":[\"http://schema.mathworks.com/mf0/Connector/R2020b\"],\"version\":\"1.0\"}"
  Subsystem4 : Subsystem
      settings: PortSchema="{\"entries\":[{\"content\":{\"sides\":[{\"content\":{\"connectorIds\":[\"In1\",\"In2\",\"In3\",\"In4\"]},\"type\":\"ConnectorPlacement.EquallySpacedRectSide\",\"uuid\":\"3c32f130-2df4-4697-80e9-267a8217898e\"},{\"content\":{\"connectorIds\":[\"Out1\"],\"side\":\"RIGHT\"},\"type\":\"ConnectorPlacement.EquallySpacedRectSide\",\"uuid\":\"840675a7-4714-440f-a6ce-75eff1b2763f\"},{\"content\":{\"connectorIds\":[\"In5\"],\"side\":\"TOP\"},\"type\":\"ConnectorPlacement.EquallySpacedRectSide\",\"uuid\":\"5c23af56-4ec3-4a39-a531-12998a0be3c8\"},{\"content\":{\"connectorIds\":[\"Out2\"],\"side\":\"BOTTOM\"},\"type\":\"ConnectorPlacement.EquallySpacedRectSide\",\"uuid\":\"31d953fb-65a0-42e9-a844-060de010f298\"}]},\"type\":\"ConnectorPlacement.EquallySpacedConnector\",\"uuid\":\"61b27aa3-5880-401e-bae3-4611093a191a\"}],\"packageUris\":[\"http://schema.mathworks.com/mf0/Connector/R2020b\"],\"version\":\"1.0\"}"
  Subsystem5 : Subsystem
      settings: PortSchema="{\"entries\":[{\"content\":{\"sides\":[{\"content\":{\"connectorIds\":[\"In1\",\"In2\",\"In3\",\"In4\"]},\"type\":\"ConnectorPlacement.EquallySpacedRectSide\",\"uuid\":\"3c32f130-2df4-4697-80e9-267a8217898e\"},{\"content\":{\"connectorIds\":[\"Out1\"],\"side\":\"RIGHT\"},\"type\":\"ConnectorPlacement.EquallySpacedRectSide\",\"uuid\":\"840675a7-4714-440f-a6ce-75eff1b2763f\"},{\"content\":{\"connectorIds\":[\"In5\"],\"side\":\"TOP\"},\"type\":\"ConnectorPlacement.EquallySpacedRectSide\",\"uuid\":\"5c23af56-4ec3-4a39-a531-12998a0be3c8\"},{\"content\":{\"connectorIds\":[\"Out2\"],\"side\":\"BOTTOM\"},\"type\":\"ConnectorPlacement.EquallySpacedRectSide\",\"uuid\":\"31d953fb-65a0-42e9-a844-060de010f298\"}]},\"type\":\"ConnectorPlacement.EquallySpacedConnector\",\"uuid\":\"61b27aa3-5880-401e-bae3-4611093a191a\"}],\"packageUris\":[\"http://schema.mathworks.com/mf0/Connector/R2020b\"],\"version\":\"1.0\"}"
  Subsystem6 : Subsystem
  Subsystem7 : Subsystem
      settings: PortSchema="{\"entries\":[{\"content\":{\"sides\":[{\"content\":{\"connectorIds\":[\"In1\",\"In2\",\"In3\",\"In4\"]},\"type\":\"ConnectorPlacement.EquallySpacedRectSide\",\"uuid\":\"3c32f130-2df4-4697-80e9-267a8217898e\"},{\"content\":{\"connectorIds\":[\"Out1\"],\"side\":\"RIGHT\"},\"type\":\"ConnectorPlacement.EquallySpacedRectSide\",\"uuid\":\"840675a7-4714-440f-a6ce-75eff1b2763f\"},{\"content\":{\"connectorIds\":[\"In5\"],\"side\":\"TOP\"},\"type\":\"ConnectorPlacement.EquallySpacedRectSide\",\"uuid\":\"5c23af56-4ec3-4a39-a531-12998a0be3c8\"},{\"content\":{\"connectorIds\":[\"Out2\"],\"side\":\"BOTTOM\"},\"type\":\"ConnectorPlacement.EquallySpacedRectSide\",\"uuid\":\"31d953fb-65a0-42e9-a844-060de010f298\"}]},\"type\":\"ConnectorPlacement.EquallySpacedConnector\",\"uuid\":\"61b27aa3-5880-401e-bae3-4611093a191a\"}],\"packageUris\":[\"http://schema.mathworks.com/mf0/Connector/R2020b\"],\"version\":\"1.0\"}"
  Subsystem8 : Subsystem
      settings: PortSchema="{\"entries\":[{\"content\":{\"sides\":[{\"content\":{\"connectorIds\":[\"In1\",\"In2\",\"In3\",\"In4\",\"In5\",\"In6\"]},\"type\":\"ConnectorPlacement.EquallySpacedRectSide\",\"uuid\":\"6e2ae49e-f829-4a88-ba6d-12a1c984ff97\"},{\"content\":{\"connectorIds\":[\"Out1\"],\"side\":\"RIGHT\"},\"type\":\"ConnectorPlacement.EquallySpacedRectSide\",\"uuid\":\"1d02df48-94d5-4b75-9fdc-37bb62799324\"},{\"content\":{\"connectorIds\":[],\"side\":\"TOP\"},\"type\":\"ConnectorPlacement.EquallySpacedRectSide\",\"uuid\":\"e0c2a01b-94eb-432a-818f-b3ac4af71c3e\"},{\"content\":{\"connectorIds\":[\"In7\"],\"side\":\"BOTTOM\"},\"type\":\"ConnectorPlacement.EquallySpacedRectSide\",\"uuid\":\"1c8c54e5-1608-4962-a210-31f0a1951aa9\"}]},\"type\":\"ConnectorPlacement.EquallySpacedConnector\",\"uuid\":\"4e183442-7783-4f10-aa1a-c21f2f9b268a\"}],\"packageUris\":[\"http://schema.mathworks.com/mf0/Connector/R2020b\"],\"version\":\"1.0\"}"
  u6 : Outport
  wires:
  Bus Creator/1 -> u6/1  "node6"
  Bus Selector/1 -> Subsystem6/1(xx6)  "<xx>"
  Bus Selector/3 -> Subsystem6/3(xx1)  "<xx>"
  Bus Selector/4 -> Subsystem6/4(xx2)  "<xx>"
  Bus Selector6/3 -> Subsystem8/6(vz)  "<vz>"
  Bus Selector6/1 -> Subsystem8/4(vx)  "<vx>"
  [Sx] -> Subsystem8/1(Sx)
  [Sz] -> Subsystem8/3(Sz)
  Subsystem8/1(" gain") -> [gain]  "p6"
  In19/1 -> [state], Bus Selector2/1, Bus Selector/1, Bus Selector1/1
  [state] -> Bus Selector6/1
  [Sy] -> Subsystem8/2(Sy)
  Bus Selector6/2 -> Subsystem8/5(vy)  "<vy>"
  Bus Selector7/3 -> Subsystem3/4(vz)  "<vz>"
  Bus Selector7/1 -> Subsystem3/2(vx)  "<vx>"
  [state] -> Bus Selector8/1
  Bus Selector8/1 -> Subsystem3/6(ux)  "<ux>"
  Bus Selector8/2 -> Subsystem3/7(uy)  "<uy>"
  Bus Selector7/2 -> Subsystem3/3(vy)  "<vy>"
  [state] -> Bus Selector7/1
  Bus Selector8/3 -> Subsystem3/8(uz)  "<uz>"
  Subsystem3/2(udty) -> Subsystem10/2(uty)
  Subsystem3/1(udtx) -> Subsystem10/1(utx)
  Subsystem3/3(udtz) -> Subsystem10/3(utz)
  Bus Selector/2 -> Subsystem6/2(xx0)  "<xx0>"
  Bus Selector/5 -> Subsystem6/5(vx6)  "<vx>"
  Bus Selector/6 -> Subsystem6/6(vx0)  "<vx0>"
  Bus Selector/7 -> Subsystem6/7(vx1)  "<vx>"
  Bus Selector/8 -> Subsystem6/8(vx2)  "<vx>"
  Bus Selector1/1 -> Subsystem1/1(xx6)  "<xy>"
  Bus Selector1/2 -> Subsystem1/2(xx0)  "<xy0>"
  Bus Selector1/3 -> Subsystem1/3(xx1)  "<xy>"
  Bus Selector1/4 -> Subsystem1/4(xx2)  "<xy>"
  Bus Selector1/5 -> Subsystem1/5(vx6)  "<vy>"
  Bus Selector1/6 -> Subsystem1/6(vx0)  "<vy0>"
  Bus Selector1/7 -> Subsystem1/7(vx1)  "<vy>"
  Bus Selector1/8 -> Subsystem1/8(vx2)  "<vy>"
  Bus Selector2/1 -> Subsystem2/1(xx6)  "<xz>"
  Bus Selector2/2 -> Subsystem2/2(xx0)  "<xz0>"
  Bus Selector2/3 -> Subsystem2/3(xx1)  "<xz>"
  Bus Selector2/4 -> Subsystem2/4(xx2)  "<xz>"
  Bus Selector2/5 -> Subsystem2/5(vx6)  "<vz>"
  Bus Selector2/6 -> Subsystem2/6(vx0)  "<vz0>"
  Bus Selector2/7 -> Subsystem2/7(vx1)  "<vz>"
  Bus Selector2/8 -> Subsystem2/8(vx2)  "<vz>"
  Subsystem4/2(Sx) -> [Sx]
  Bus Selector5/2 -> Subsystem7/2(vz0)  "<vz>"
  Subsystem5/2(Sz) -> [Sy]
  Subsystem7/2(Sz) -> [Sz]
  [gain] -> Subsystem5/4(gain)
  [state] -> Bus Selector3/1
  Bus Selector5/1 -> Subsystem7/1(vz6)  "<vz>"
  Bus Selector4/2 -> Subsystem5/2(vy0)  "<vx>"
  [gain] -> Subsystem4/4(gain)
  [state] -> Bus Selector5/1
  Subsystem7/1(uz) -> Subsystem3/9(utz)
  Subsystem5/1(uy) -> Subsystem3/5(uty)
  Subsystem4/1(ux) -> Subsystem3/1(utx)
  Bus Selector3/1 -> Subsystem4/1(vx6)  "<vx>"
  Bus Selector3/2 -> Subsystem4/2(vx0)  "<vx>"
  [gain] -> Subsystem7/4(gain)
  [state] -> Bus Selector4/1
  Bus Selector4/1 -> Subsystem5/1(vy6)  "<vy>"
  [switch] -> Subsystem5/5(switch)
  [switch] -> Subsystem7/5(switch)
  Subsystem6/1(utx) -> Subsystem4/3(utx)
  Subsystem1/1(utx) -> Subsystem5/3(uty)
  Subsystem2/1(utx) -> Subsystem7/3(utz)
  switch/1 -> [switch], Subsystem4/5(switch)
  [switch] -> Subsystem8/7(switch)
  [switch] -> Subsystem3/10(switch)
  Subsystem10/2(uy) -> Bus Creator/2  "uy"
  Subsystem10/3(uz) -> Bus Creator/3  "uz"
  Subsystem10/1(ux) -> Bus Creator/1  "ux"
